simulink model "traj_test"  (R2023b)
settings: Solver=ode1  StartTime=0.0  StopTime=170  FixedStep=Ts  RelTol=1e-3
values from neighbouring files (symbols this model uses):
  q0 = [0, -0.60, 0, -2.25, 0, 1.5, 0.8]'    [Panda_run.m]
  q1 = traj_c.qd.Data(:,1,1)    [Panda_run.m]
settings Model: Creator=robot102  LastModifiedBy=robot102

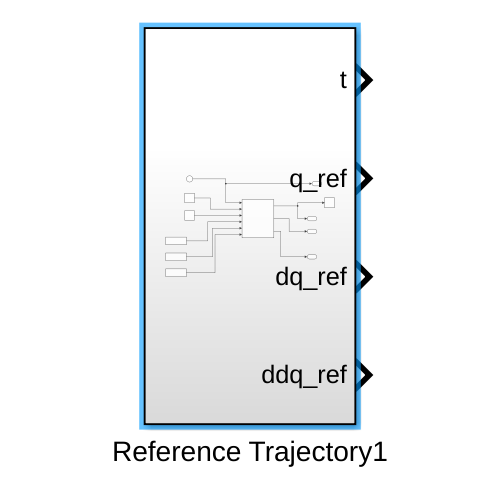
[thumbnail: Simulink's stored preview of the top-level diagram]
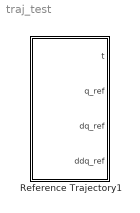
== system traj_test ==
  Reference Trajectory1 : Subsystem

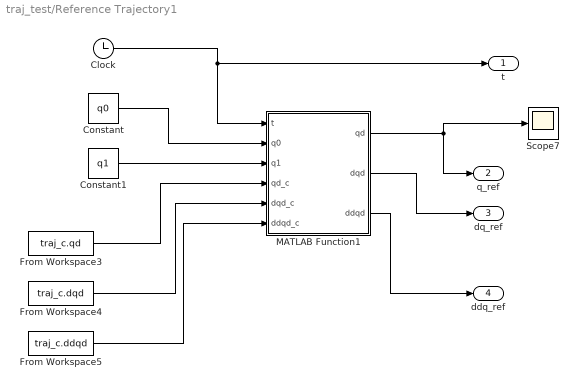
== system traj_test/Reference Trajectory1 ==
  Clock : Clock
  Constant : Constant  Value=q0
  Constant1 : Constant  Value=q1
  From Workspace3 : FromWorkspace  VariableName=traj_c.qd
  From Workspace4 : FromWorkspace  VariableName=traj_c.dqd
  From Workspace5 : FromWorkspace  VariableName=traj_c.ddqd
  MATLAB Function1 : MATLAB Function  TreatAsAtomicUnit=on
  Scope7 : Scope
  t : Outport
  q_ref : Outport  Port=2
  dq_ref : Outport  Port=3
  ddq_ref : Outport  Port=4
  wires:
  MATLAB Function1/1(qd) -> q_ref/1, Scope7/1
  MATLAB Function1/2(dqd) -> dq_ref/1
  MATLAB Function1/3(ddqd) -> ddq_ref/1
  From Workspace3/1 -> MATLAB Function1/4(qd_c)
  From Workspace4/1 -> MATLAB Function1/5(dqd_c)
  From Workspace5/1 -> MATLAB Function1/6(ddqd_c)
  Clock/1 -> MATLAB Function1/1(t), t/1
  Constant/1 -> MATLAB Function1/2(q0)
  Constant1/1 -> MATLAB Function1/3(q1)

== matlab function traj_test/Reference Trajectory1/MATLAB Function1 ==
  data: t input; q0 input; q1 input; qd output; dqd output; ddqd output; qd_c input; dqd_c input; ddqd_c input
function [qd,dqd,ddqd] = fcn(t,q0,q1,qd_c,dqd_c,ddqd_c)

if t<=100
    T=[0,3,6,9,13,17,20,23];
    P=[q0';
        -0.75, 0.25, 0, -0.8, -1.2, 0.5, -1.8;
        1.5, 0.6, -0.83, -0.5, 1.04, 1.6, -2.0;
        0.25, -0.55, 0.3, -1.75, 0.25, 0.75, 0.50;
        -1.20, 0.84, -0.85, -1.0, 1.07, 2.55, 2.05;
        -2.25, -1.2, 2.23, -0.63, -0.54, 2.8, 1.3;
        -0.25, 1.0, -0.23, -1.33, -0.24, 1.1, -2.5;
        q0'];
    [qd,dqd,ddqd]=traj_gen_fun(t,T,P);
elseif t<=120
    T=[100,105];
    P=[q0,q1]';
    [qd,dqd,ddqd]=traj_gen_fun(t,T,P);
elseif t<=160
    qd=qd_c;dqd=dqd_c;ddqd=ddqd_c;
else
    T=[160,165];
    P=[q1,q0]';
    [qd,dqd,ddqd]=traj_gen_fun(t,T,P);

    % qd=[0, -0.60, 0, -2.25, 0, 1.5, 0.8]';
    % dqd=zeros(7,1);
    % ddqd=zeros(7,1);
end
